simulink model "test"  (R2014b)
settings: Solver=ode45  StartTime=0.0  StopTime=1  RelTol=1e-3
undefined symbols (not defined in the file or in its folder): SLIF_Frame, SLIF_PSF_SampPerSym, SLIF_Rsymbol
libraries: commrandsrc2 x1, commdigbbndfm2 x1, dspsrcs4 x1
settings Model: Creator=Ben  LastModifiedBy=Ben

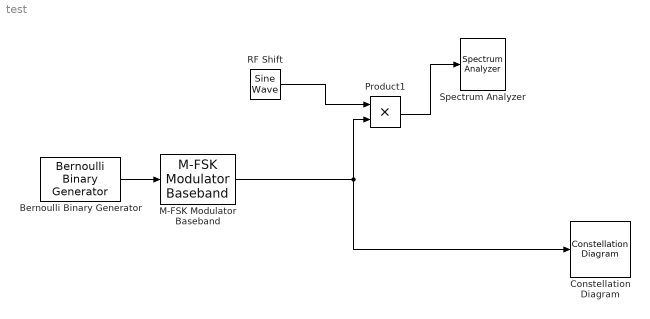
== system test ==
  Bernoulli Binary Generator : commrandsrc2/Bernoulli Binary Generator  P=0.5  seed=11  Ts=1/SLIF_Rsymbol  frameBased=on  sampPerFrame=SLIF_Frame  orient=off  outDataType=double
  Constellation Diagram : ConstellationDiagram
  M-FSK Modulator Baseband : commdigbbndfm2/M-FSK Modulator Baseband  M=2  InType=Integer  Enc=Binary  freqSep=pi/2  phaseType=Continuous  numSamp=SLIF_PSF_SampPerSym  RateOptions=Enforce single-rate processing  outDataType=double
  Product1 : Product  RndMeth=Zero
  RF Shift : dspsrcs4/Sine Wave  Amplitude=2  Frequency=1000000  Phase=0  SampleMode=Discrete  OutComplex=Complex  CompMethod=Trigonometric fcn  TableSize=Speed  SampleTime=1/(SLIF_Rsymbol*SLIF_PSF_SampPerSym)  SamplesPerFrame=SLIF_PSF_SampPerSym*SLIF_Frame  ResetState=Restart at time zero  dataType=double  wordLen=16  udDataType=sfix(16)  fracBitsMode=Best precision  numFracBits=15  OutDataTypeStr=double  LastOutDataTypeStr=double
  Spectrum Analyzer : SpectrumAnalyzer
  wires:
  Bernoulli Binary Generator/1 -> M-FSK Modulator Baseband/1
  RF Shift/1 -> Product1/1
  M-FSK Modulator Baseband/1 -> Product1/2, Constellation Diagram/1
  Product1/1 -> Spectrum Analyzer/1
